simulink model "Zustandsregelung_mit_I_Regelung_linear"  (R2021b)
settings: Solver=FixedStepAuto  StartTime=0.0  StopTime=25  FixedStep=1/1e4  RelTol=1e-3
values from neighbouring files (symbols this model uses):
  A = double(subs(A, {x(1), x(2), x(3), x(4)}, {xRuhe(1), xRuhe(2), xRuhe(3), xRuhe(4)}))    [Lineares_Zustandsraummodell.m]
  B = double(subs(B, {x(1), x(2), x(3), x(4)}, {xRuhe(1), xRuhe(2), xRuhe(3), xRuhe(4)}))    [Lineares_Zustandsraummodell.m]
  C_I_Regelung = [0 0 1 0]    [Main.m]
undefined symbols (not defined in the file or in its folder): start_deg, y_ref
settings Model: Creator=basti  LastModifiedBy=aaron

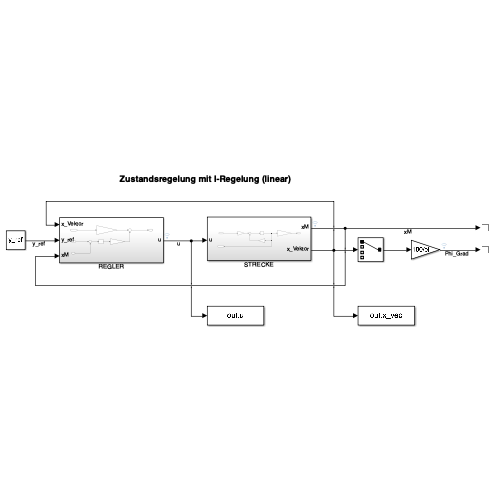
[thumbnail: Simulink's stored preview of the top-level diagram]
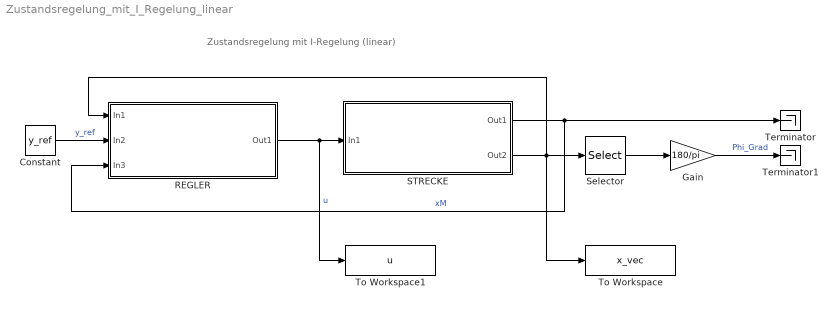
== system Zustandsregelung_mit_I_Regelung_linear ==
  note: Zustandsregelung mit I-Regelung (linear)
  Constant : Constant  Value=y_ref
  Gain : Gain  Gain=180/pi
  REGLER : Subsystem
  STRECKE : Subsystem
  Selector : Selector  InputPortWidth=4  IndexOptions=Index vector (dialog)  Indices=1  OutputSizes=1
  Terminator : Terminator
  Terminator1 : Terminator
  To Workspace : ToWorkspace  VariableName=x_vec  SaveFormat=Timeseries  SampleTime=-1
  To Workspace1 : ToWorkspace  VariableName=u  SaveFormat=Timeseries  SampleTime=-1
  wires:
  STRECKE/1(Out1) -> Terminator/1, REGLER/3(In3)  "xM"
  Constant/1 -> REGLER/2(In2)  "y_ref"
  STRECKE/2(Out2) -> To Workspace/1, Selector/1, REGLER/1(In1)
  REGLER/1(Out1) -> To Workspace1/1, STRECKE/1(In1)  "u"
  Selector/1 -> Gain/1
  Gain/1 -> Terminator1/1  "Phi_Grad"

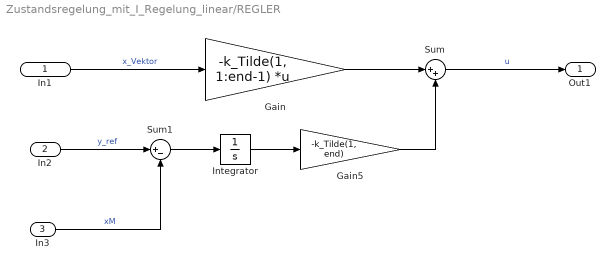
== system Zustandsregelung_mit_I_Regelung_linear/REGLER ==
  In1 : Inport
  In2 : Inport  Port=2
  In3 : Inport  Port=3
  Gain : Gain  Gain=-k_Tilde(1, 1:end-1)  Multiplication=Matrix(K*u) (u vector)
  Gain5 : Gain  Gain=-k_Tilde(1, end)
  Integrator : Integrator
  Sum : Sum  Inputs=|++
  Sum1 : Sum  Inputs=|+-
  Out1 : Outport
  wires:
  Gain/1 -> Sum/1
  In1/1 -> Gain/1  "x_Vektor"
  Sum/1 -> Out1/1  "u"
  In2/1 -> Sum1/1  "y_ref"
  In3/1 -> Sum1/2  "xM"
  Integrator/1 -> Gain5/1
  Sum1/1 -> Integrator/1
  Gain5/1 -> Sum/2

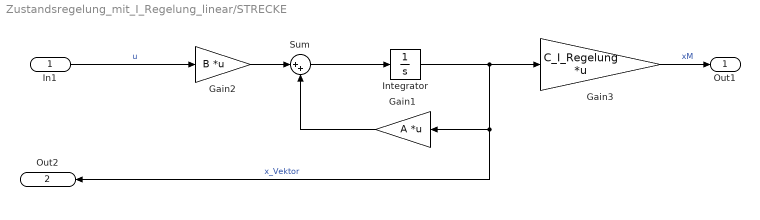
== system Zustandsregelung_mit_I_Regelung_linear/STRECKE ==
  In1 : Inport
  Gain1 : Gain  Gain=A  Multiplication=Matrix(K*u) (u vector)
  Gain2 : Gain  Gain=B  Multiplication=Matrix(K*u) (u vector)
  Gain3 : Gain  Gain=C_I_Regelung  Multiplication=Matrix(K*u) (u vector)
  Integrator : Integrator  InitialCondition=[(start_deg*pi)/180 0 0 0]
  Sum : Sum  Inputs=|++
  Out1 : Outport
  Out2 : Outport  Port=2
  wires:
  Gain1/1 -> Sum/2
  Gain3/1 -> Out1/1  "xM"
  Sum/1 -> Integrator/1
  Integrator/1 -> Out2/1, Gain1/1, Gain3/1  "x_Vektor"
  Gain2/1 -> Sum/1
  In1/1 -> Gain2/1  "u"
